simulink model "Model"  (R2024b)
settings: Solver=ode45  StartTime=0.0  StopTime=3  FixedStep=0.001  RelTol=1e-3
InitFcn:
  | Main
values from neighbouring files (symbols this model uses):
  A = [0, 1; 0, -20]    [Main.m]
  Ao = Ae - L*Ce    [Main.m]
  B = [0; 60]    [Main.m]
  Bo = [Be, L]    [Main.m]
  C = [1, 0]    [Main.m]
  Co = eye(5)    [Main.m]
  Cp = [1, 0, 0]    [Main.m]
  D = 0    [Main.m]
  Do = zeros(5, 2)    [Main.m]
  K = place(A, B, Lc)    [Main.m]
  W = 6    [Main.m]
settings Model: Creator=Banaan  LastModifiedBy=Banaan

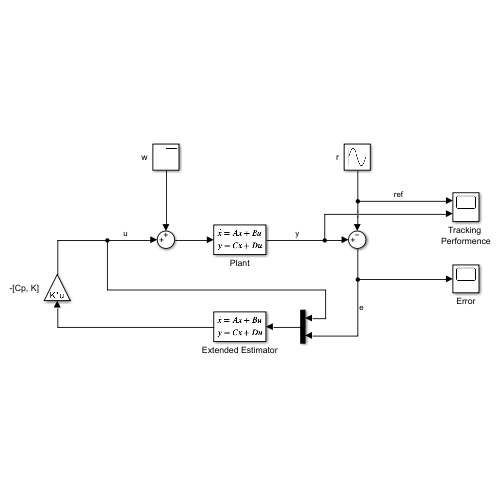
[thumbnail: Simulink's stored preview of the top-level diagram]
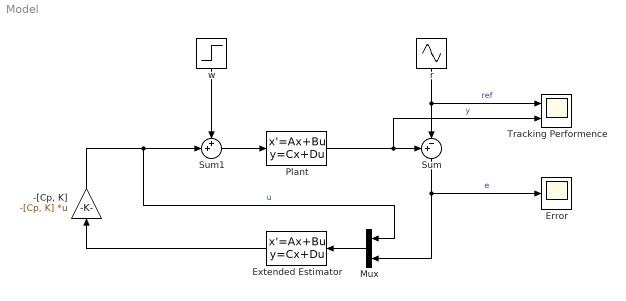
== system Model ==
  "-[Cp, K]" : Gain  Gain=-[Cp, K]  Multiplication=Matrix(K*u)
  Error : Scope
  Extended Estimator : StateSpace  A=Ao  B=Bo  C=Co  D=Do  InitialCondition=0
  Mux : Mux  Inputs=2
  Plant : StateSpace  A=A  B=B  C=C  D=D  InitialCondition=0
  Sum : Sum  Inputs=+-|
  Sum1 : Sum  Inputs=++|
  Tracking Performence : Scope  NumInputPorts=2
  r : Sin  Frequency=W  SampleTime=0
  w : Step  SampleTime=0
  wires:
  Mux/1 -> Extended Estimator/1
  Extended Estimator/1 -> "-[Cp, K]"/1
  Plant/1 -> Tracking Performence/2, Sum/1  "y"
  Sum/1 -> Error/1, Mux/2  "e"
  w/1 -> Sum1/1
  Sum1/1 -> Plant/1
  r/1 -> Tracking Performence/1, Sum/2  "ref"
  "-[Cp, K]"/1 -> Mux/1, Sum1/2  "u"
